simulink model "modelo_n_linear0_1"  (R2013a)
settings: Solver=ode45  StartTime=0.0  StopTime=0.5  RelTol=1e-3
values from neighbouring files (symbols this model uses):
  Fp_model = fit_Kb    [parametriza.m]
  gb = 0.3e-3    (= 0.0003)    [parametriza.m]    (also in parametrizaMancal.m)
  gi = 0.7e-3    (= 0.0007)    [parametriza.m]    (also in parametrizaMancal.m)
  K1 = u0/Sg    (= 0.00637886833216)    [parametriza.m]
  K2 = 1/u0/N    (= 2652.58238486)    [parametriza.m]
  Kp = 625    [parametriza.m]
  L1 = -1.206e-05    [parametriza.m]
  L2 = 7.807e-05    [parametriza.m]
  m = 0.375    [parametriza.m]    (also in parametrizaMancal.m)
  R = 6.3    [parametriza.m]    (also in parametrizaMancal.m = 6)
libraries: simulink x1
settings Model: Creator=rafa  LastModifiedBy=rafa

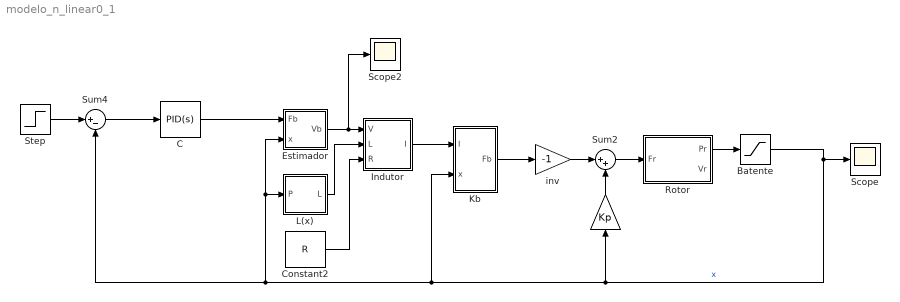
== system modelo_n_linear0_1 ==
  " " : Gain  Gain=Kp
  Batente : Saturate  UpperLimit=gb  LowerLimit=-gb
  C : simulink/Continuous/PID Controller  Controller=PID  TimeDomain=Continuous-time  SampleTime=1  IntegratorMethod=Forward Euler  FilterMethod=Forward Euler  Form=Ideal  P=-20745.2608556977  I=5.69123962803468  D=0.0177336811288622  N=1559.20264332968  InitialConditionSource=internal  InitialConditionForIntegrator=0  InitialConditionForFilter=0  ExternalReset=none  LimitOutput=off  UpperSaturationLimit=inf  LowerSaturationLimit=-inf  LinearizeAsGain=on  AntiWindupMode=none  Kb=1  TrackingMode=off  Kt=1  PParamMin=[]  PParamMax=[]  IParamMin=[]  IParamMax=[]  DParamMin=[]  DParamMax=[]  NParamMin=[]  NParamMax=[]  KbParamMin=[]  KbParamMax=[]  KtParamMin=[]  KtParamMax=[]  POutMin=[]  POutMax=[]  IOutMin=[]  IOutMax=[]  DOutMin=[]  DOutMax=[]  NOutMin=[]  NOutMax=[]  KbOutMin=[]  KbOutMax=[]  KtOutMin=[]  KtOutMax=[]  IntegratorOutMin=[]  IntegratorOutMax=[]  FilterOutMin=[]  FilterOutMax=[]  SumOutMin=[]  SumOutMax=[]  SumI1OutMin=[]  SumI1OutMax=[]  SumI2OutMin=[]  SumI2OutMax=[]  SumI3OutMin=[]  SumI3OutMax=[]  SumDOutMin=[]  SumDOutMax=[]  SaturationOutMin=[]  SaturationOutMax=[]  IntegratorContinuousStateAttributes=''  IntegratorStateMustResolveToSignalObject=off  IntegratorRTWStateStorageClass=Auto  FilterContinuousStateAttributes=''  FilterStateMustResolveToSignalObject=off  FilterRTWStateStorageClass=Auto
  Constant2 : Constant  Value=R
  Estimador : Subsystem
  Indutor : Subsystem
  Kb : Subsystem
  L(x) : Subsystem
  Rotor : Subsystem
  Scope : Scope
      settings: YMin=9.75e-05  YMax=0.0001525  SaveName=simulink_posicao
  Scope2 : Scope
      settings: YMin=9.75e-05  YMax=0.0001525  SaveName=simulink_esforco
  Step : Step  Time=0  After=0  SampleTime=0
  Sum2 : Sum  Inputs=|++
  Sum4 : Sum  Inputs=|+-
  inv : Gain  Gain=-1
  wires:
  L(x)/1(L) -> Indutor/2(L)
  Constant2/1 -> Indutor/3(R)
  Indutor/1(I) -> Kb/1(I)
  Kb/1(Fb) -> inv/1
  inv/1 -> Sum2/1
  " "/1 -> Sum2/2
  Sum2/1 -> Rotor/1(Fr)
  Sum4/1 -> C/1
  Step/1 -> Sum4/1
  Batente/1 -> Scope/1, " "/1, Kb/2(x), Estimador/2(x), L(x)/1(P), Sum4/2  "x"
  Estimador/1(Vb) -> Scope2/1, Indutor/1(V)
  Rotor/1(Pr) -> Batente/1
  C/1 -> Estimador/1("Fb ")

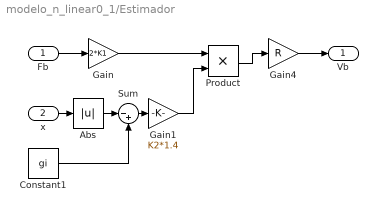
== system modelo_n_linear0_1/Estimador ==
  "Fb " : Inport
  x : Inport  Port=2
  Abs : Abs
  Constant1 : Constant  Value=gi
  Gain : Gain  Gain=2*K1
  Gain1 : Gain  Gain=K2*1.4
  Gain4 : Gain  Gain=R
  Product : Product
  Sum : Sum  Inputs=|-+
  Vb : Outport
  wires:
  Gain4/1 -> Vb/1
  "Fb "/1 -> Gain/1
  Gain/1 -> Product/1
  Product/1 -> Gain4/1
  Abs/1 -> Sum/1
  x/1 -> Abs/1
  Constant1/1 -> Sum/2
  Sum/1 -> Gain1/1
  Gain1/1 -> Product/2

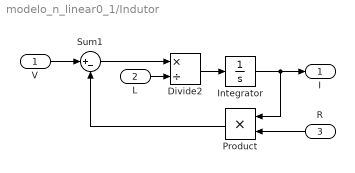
== system modelo_n_linear0_1/Indutor ==
  V : Inport
  L : Inport  Port=2
  R : Inport  Port=3
  Divide2 : Product  Inputs=*/
  Integrator : Integrator
  Product : Product
  Sum1 : Sum  Inputs=|+-
  I : Outport
  wires:
  Divide2/1 -> Integrator/1
  Sum1/1 -> Divide2/1
  Integrator/1 -> Product/1, I/1
  Product/1 -> Sum1/2
  L/1 -> Divide2/2
  V/1 -> Sum1/1
  R/1 -> Product/2

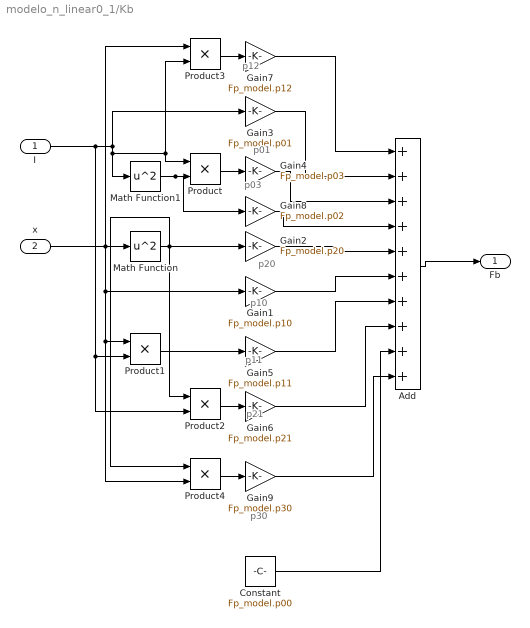
== system modelo_n_linear0_1/Kb ==
  note: p12
  note: p01
  note: p20
  note: p10
  note: p11
  note: p21
  note: p30
  note: p03
  I : Inport
  x : Inport  Port=2
  Add : Sum  Inputs=++++++++++
  Constant : Constant  Value=Fp_model.p00
  Gain1 : Gain  Gain=Fp_model.p10
  Gain2 : Gain  Gain=Fp_model.p20
  Gain3 : Gain  Gain=Fp_model.p01
  Gain4 : Gain  Gain=Fp_model.p03
  Gain5 : Gain  Gain=Fp_model.p11
  Gain6 : Gain  Gain=Fp_model.p21
  Gain7 : Gain  Gain=Fp_model.p12
  Gain8 : Gain  Gain=Fp_model.p02
  Gain9 : Gain  Gain=Fp_model.p30
  Math Function : Math  Operator=square  SaturateOnIntegerOverflow=on
  Math Function1 : Math  Operator=square  SaturateOnIntegerOverflow=on
  Product{,1..4} (5 alike) : Product  RndMeth=Zero
  Fb : Outport
  wires:
  I/1 -> Product2/2, Product1/2, Gain3/1, Math Function1/1, Product/1, Product3/2
  Product/1 -> Gain4/1
  Math Function1/1 -> Gain8/1, Product/2
  Gain4/1 -> Add/3
  x/1 -> Product3/1, Product4/2, Product1/1, Gain1/1, Math Function/1
  Math Function/1 -> Product4/1, Product2/1, Gain2/1
  Product1/1 -> Gain5/1
  Product2/1 -> Gain6/1
  Product3/1 -> Gain7/1
  Constant/1 -> Add/9
  Gain7/1 -> Add/1
  Gain3/1 -> Add/2
  Gain8/1 -> Add/4
  Gain2/1 -> Add/5
  Gain1/1 -> Add/6
  Gain5/1 -> Add/7
  Gain6/1 -> Add/8
  Add/1 -> Fb/1
  Product4/1 -> Gain9/1
  Gain9/1 -> Add/10

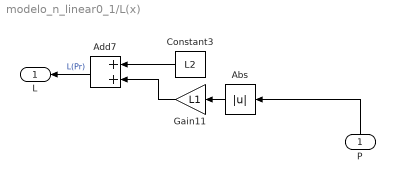
== system modelo_n_linear0_1/L(x) ==
  P : Inport
  Abs : Abs
  Add7 : Sum
  Constant3 : Constant  Value=L2
  Gain11 : Gain  Gain=L1
  L : Outport
  wires:
  P/1 -> Abs/1
  Add7/1 -> L/1  "L(Pr)"
  Constant3/1 -> Add7/1
  Gain11/1 -> Add7/2
  Abs/1 -> Gain11/1

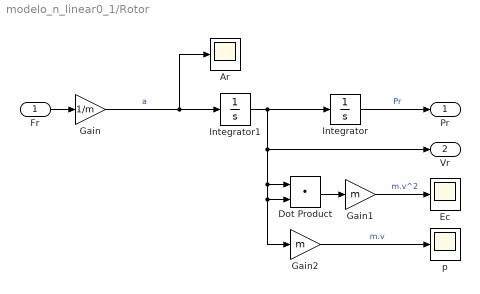
== system modelo_n_linear0_1/Rotor ==
  Fr : Inport
  Ar : Scope
      settings: TimeRange=1  YMin=-200000  YMax=200000  SaveName=ScopeData9
  Dot Product : DotProduct  InputSameDT=on  OutDataTypeStr=Inherit: Inherit via internal rule
  Ec : Scope
      settings: TimeRange=0.25  YMin=0  YMax=0.09  SaveName=ScopeData16
  Gain : Gain  Gain=1/m
  Gain1 : Gain  Gain=m
  Gain2 : Gain  Gain=m
  Integrator : Integrator  UpperSaturationLimit=Inf  LowerSaturationLimit=-Inf
  Integrator1 : Integrator
  p : Scope
      settings: TimeRange=1  YMin=-200000  YMax=200000  SaveName=ScopeData17
  Pr : Outport
  Vr : Outport  Port=2
  wires:
  Fr/1 -> Gain/1
  Integrator/1 -> Pr/1  "Pr"
  Gain/1 -> Ar/1, Integrator1/1  "a"
  Dot Product/1 -> Gain1/1
  Gain2/1 -> p/1  "m.v"
  Gain1/1 -> Ec/1  "m.v^2"
  Integrator1/1 -> Vr/1, Dot Product/1, Gain2/1, Dot Product/2, Integrator/1
